simulink model "scatteredInterpolant_model"  (R2026a)
settings: Solver=FixedStepDiscrete  StopTime=tFinal_s  FixedStep=deltaT_s
values from neighbouring files (symbols this model uses):
  alt_initial_output_kft = 0    [demo_scatteredInterpolant.m]
  alt_slope_kftps = max(alt_vec_kft) - min(alt_vec_kft)    [demo_scatteredInterpolant.m]
  alt_vec_kft = linspace(min(alt_kft)-Ly*envelopeExpansionFactor,max(alt_kft)+Ly*envelopeExpansionFactor,35)    [demo_scatteredInterpolant.m]
  mach_initial_output = 0.8    [demo_scatteredInterpolant.m]
  mach_slope = 0    [demo_scatteredInterpolant.m]
  mach_vec = linspace(min(mach)-Lx*envelopeExpansionFactor,max(mach)+Lx*envelopeExpansionFactor,25)    [demo_scatteredInterpolant.m]
  maxTurn_mesh_g = interpolant(mach_mesh,alt_mesh_kft)    [demo_scatteredInterpolant.m]
libraries: simulink x2
settings Model: Creator=chris  LastModifiedBy=chris

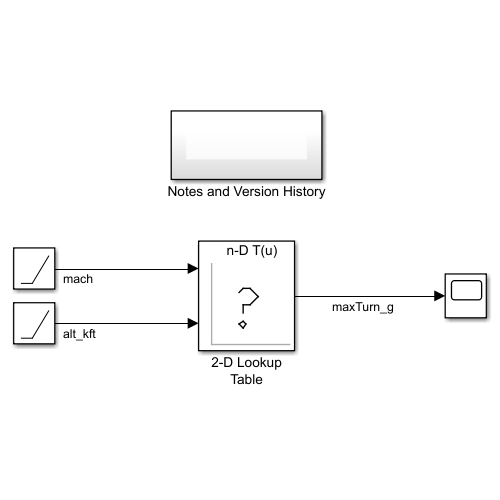
[thumbnail: Simulink's stored preview of the top-level diagram]
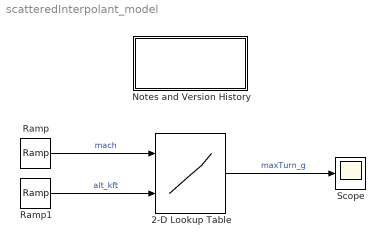
== system scatteredInterpolant_model ==
  2-D Lookup Table : Lookup_n-D  BreakpointsForDimension1=mach_vec  BreakpointsForDimension2=alt_vec_kft  Table=maxTurn_mesh_g  InternalRulePriority=Speed  RndMeth=Simplest
      settings: InputPortMap=u0,u1
  Notes and Version History : Subsystem
  Ramp : simulink/Sources/Ramp  slope=mach_slope  start=0  InitialOutput=mach_initial_output
  Ramp1 : simulink/Sources/Ramp  slope=alt_slope_kftps  start=0  InitialOutput=alt_initial_output_kft
  Scope : Scope
  wires:
  Ramp/1 -> 2-D Lookup Table/1  "mach"
  Ramp1/1 -> 2-D Lookup Table/2  "alt_kft"
  2-D Lookup Table/1 -> Scope/1  "maxTurn_g"

== system scatteredInterpolant_model/Notes and Version History ==
  note: Demonstrate using a lookup table (data was generated using scatteredInterpolant)
      |
      | Christohper Lum
      | lum@uw.edu
      |
      | Version History
      | 10/04/26: Created
